simulink library "Uav_Electrical_lib"  (R2025a)
settings: Solver=ode23t  StartTime=0.0  StopTime=10  MaxStep=1e-3  RelTol=1e-3
values from neighbouring files (symbols this model uses):
  Ts = 2e-6    (= 2e-06)    [param.m]
undefined symbols (not defined in the file or in its folder): DiscIntNeverNeededParam, magnitude, uavParams
libraries: fl_lib x118, nesl_utility x61, spsCurrentMeasurementLib x23, spsIdealSwitchLib x12, spsVoltageMeasurementLib x11, simulink_extras x8, spsControlledCurrentSourceLib x7, spsSeriesRLCBranchLib x6, simulink x6, spsControlledVoltageSourceLib x5, spsPermanentMagnetSynchronousMachineLib x4, ee_lib x4
(part 2 of 5)

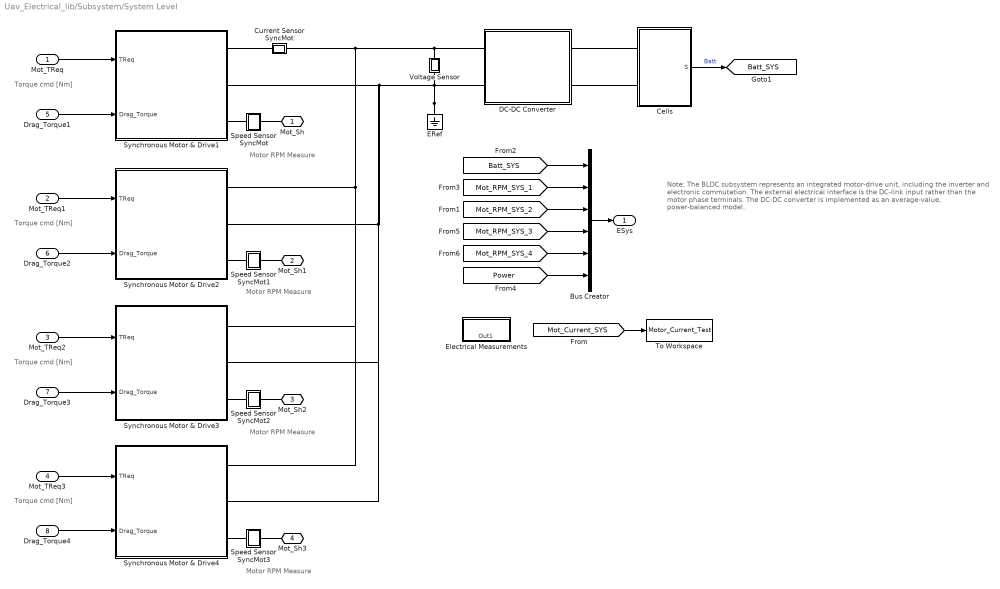
== system Uav_Electrical_lib/Subsystem/System Level ==
  note: Note:
      | The BLDC subsystem represents an integrated motor-drive unit, including the inverter and electronic commutation. The external electrical interface is the DC-link input rather than the motor phase terminals.
      |
      | The DC-DC converter is implemented as an average-value, power-balanced model.
  note: Motor RPM Measure
  note: Torque cmd [Nm]
  note: Motor RPM Measure
  note: Motor RPM Measure
  note: Motor RPM Measure
  note: Torque cmd [Nm]
  note: Torque cmd [Nm]
  note: Torque cmd [Nm]
  Mot_TReq : Inport
  Mot_TReq1 : Inport  Port=2
  Mot_TReq2 : Inport  Port=3
  Mot_TReq3 : Inport  Port=4
  Drag_Torque1 : Inport  Port=5
  Drag_Torque2 : Inport  Port=6
  Drag_Torque3 : Inport  Port=7
  Drag_Torque4 : Inport  Port=8
  Bus Creator : BusCreator  Inputs=6
  Cells : Subsystem
      mask Display:
      | port_label('LConn',1,'+');
      | port_label('LConn',2,'-');
      | port_label('output',1,'S');
  Current Sensor SyncMot : Subsystem
  DC-DC Converter : Subsystem  mask{Vout=uavParams.DCDCConv.Output_Voltage, RLoadLoss=uavParams.DCDCConv.Resistance_Losses, Kp=uavParams.DCDCConv.Kp, Ki=uavParams.DCDCConv.Ki}
      mask prompts: Vout "Output Voltage (V)"; RLoadLoss "Resistance, Load Dependent Losses (Ohm)"; Kp "Proportional Gain"; Ki "Integral Gain"
      mask Display:
      | port_label('RConn',1,'Bus+');
      | port_label('RConn',2,'Bus-');
      | port_label('LConn',1,'Batt+');
      | port_label('LConn',2,'Batt-');
      | text(0.05,0.5,'Out');
      | text(0.85,0.5,'In');
      | text(0.4,0.925,'Loss');
  ERef : fl_lib/Electrical/Electrical Elements/Electrical Reference
  Electrical Measurements : Subsystem
      settings: PortSchema="{\"entries\":[{\"content\":{\"sides\":[{\"content\":{},\"type\":\"ConnectorPlacement.EquallySpacedRectSide\",\"uuid\":\"d767dc0f-3242-457c-b485-d2cffe9a551f\"},{\"content\":{\"side\":\"RIGHT\"},\"type\":\"ConnectorPlacement.EquallySpacedRectSide\",\"uuid\":\"af281f4d-1d90-4252-9345-da5138a7006e\"},{\"content\":{\"side\":\"TOP\"},\"type\":\"ConnectorPlacement.EquallySpacedRectSide\",\"uuid\":\"dbc22d34-bfc6-4c39-8948-88a84cca37c4\"},{\"content\":{\"connectorIds\":[\"Out1\"],\"side\":\"BOTTOM\"},\"type\":\"ConnectorPlacement.EquallySpacedRectSide\",\"uuid\":\"dcc551d0-4ea4-47a9-a013-a7fbdb3e3c88\"}]},\"type\":\"ConnectorPlacement.EquallySpacedConnector\",\"uuid\":\"b183f40c-b7db-4954-8a30-0f5d22085f86\"}],\"packageUris\":[\"http://schema.mathworks.com/mf0/Connector/R2020b\"],\"version\":\"1.0\"}"
  Speed Sensor SyncMot : Subsystem
      mask Display: disp('S');
  Speed Sensor SyncMot1 : Subsystem
      mask Display: disp('S');
  Speed Sensor SyncMot2 : Subsystem
      mask Display: disp('S');
  Speed Sensor SyncMot3 : Subsystem
      mask Display: disp('S');
  Synchronous Motor & Drive1 : Subsystem
  Synchronous Motor & Drive2 : Subsystem
  Synchronous Motor & Drive3 : Subsystem
  Synchronous Motor & Drive4 : Subsystem
  To Workspace : ToWorkspace  VariableName=Motor_Current_Test  SaveFormat=Timeseries  SampleTime=-1
  Voltage Sensor : Subsystem
  Mot_Sh : PMIOPort  Side=Right
  Mot_Sh1 : PMIOPort  Port=2  Side=Right
  Mot_Sh2 : PMIOPort  Port=3  Side=Right
  Mot_Sh3 : PMIOPort  Port=4  Side=Right
  ESys : Outport  VectorParamsAs1DForOutWhenUnconnected=off
  tag scope: Batt_SYS=global
  wires:
  Bus Creator/1 -> ESys/1
  [Mot_RPM_SYS_1] -> Bus Creator/2
  Mot_TReq/1 -> Synchronous Motor & Drive1/1(TReq)
  Mot_TReq1/1 -> Synchronous Motor & Drive2/1(TReq)
  Mot_TReq2/1 -> Synchronous Motor & Drive3/1(TReq)
  Mot_TReq3/1 -> Synchronous Motor & Drive4/1(TReq)
  [Batt_SYS] -> Bus Creator/1
  Cells/1(S) -> [Batt_SYS]  "Batt"
  [Power] -> Bus Creator/6
  [Mot_RPM_SYS_4] -> Bus Creator/5
  [Mot_RPM_SYS_3] -> Bus Creator/4
  [Mot_RPM_SYS_2] -> Bus Creator/3
  [Mot_Current_SYS] -> To Workspace/1
  Drag_Torque1/1 -> Synchronous Motor & Drive1/2(Drag_Torque)
  Drag_Torque2/1 -> Synchronous Motor & Drive2/2(Drag_Torque)
  Drag_Torque3/1 -> Synchronous Motor & Drive3/2(Drag_Torque)
  Drag_Torque4/1 -> Synchronous Motor & Drive4/2(Drag_Torque)
  connections:
  Mot_Sh/RConn1 -- Speed Sensor SyncMot/RConn1
  Current Sensor SyncMot/RConn1 -- Synchronous Motor & Drive1/RConn1
  Speed Sensor SyncMot/LConn1 -- Synchronous Motor & Drive1/RConn3
  Mot_Sh1/RConn1 -- Speed Sensor SyncMot1/RConn1
  Synchronous Motor & Drive2/RConn3 -- Speed Sensor SyncMot1/LConn1
  Speed Sensor SyncMot2/LConn1 -- Synchronous Motor & Drive3/RConn3
  Mot_Sh2/RConn1 -- Speed Sensor SyncMot2/RConn1
  Mot_Sh3/RConn1 -- Speed Sensor SyncMot3/RConn1
  Speed Sensor SyncMot3/LConn1 -- Synchronous Motor & Drive4/RConn3
  Cells/LConn1 -- DC-DC Converter/LConn1
  Cells/LConn2 -- DC-DC Converter/LConn2
  Current Sensor SyncMot/LConn1 -- Synchronous Motor & Drive4/RConn1 -- Synchronous Motor & Drive3/RConn1 -- Synchronous Motor & Drive2/RConn1 -- DC-DC Converter/RConn1 -- Voltage Sensor/LConn1
  ERef/LConn1 -- Synchronous Motor & Drive3/RConn2 -- Synchronous Motor & Drive4/RConn2 -- Synchronous Motor & Drive2/RConn2 -- Synchronous Motor & Drive1/RConn2 -- DC-DC Converter/RConn2 -- Voltage Sensor/RConn1

== system Uav_Electrical_lib/Detailed （on-going work）/DC//DC Converter/PWM ==
  Ref. : Inport
  Data Type Conversion : DataTypeConversion
  Data Type Conversion1 : DataTypeConversion
  Mux : Mux  Inputs=2
  NOT : Logic  Operator=NOT  Inputs=1  AllPortsSameDT=off  OutDataTypeStr=uint(8)
  Rate Transition : RateTransition
  Relational Operator : RelationalOperator  Operator=>  InputSameDT=off
  Sawtooth generator : Subsystem
  Thermal Model : Subsystem
  Zero-Order Hold : ZeroOrderHold  SampleTime=Ts
  Pulses : Outport  VectorParamsAs1DForOutWhenUnconnected=off
  wires:
  NOT/1 -> Mux/2
  Rate Transition/1 -> Zero-Order Hold/1
  Relational Operator/1 -> Data Type Conversion/1
  Data Type Conversion/1 -> Mux/1, NOT/1
  Zero-Order Hold/1 -> Relational Operator/1
  Sawtooth generator/1(Out) -> Relational Operator/2
  Ref./1 -> Rate Transition/1, Thermal Model/1(IBus)
  Mux/1 -> Data Type Conversion1/1
  Data Type Conversion1/1 -> Pulses/1

== system Uav_Electrical_lib/Detailed （on-going work）/DC//DC Converter/Voltage Controller ==
  Uref : Inport
  UBus : Inport  Port=2
  Clock1 : Clock
  Compare To Constant1 : simulink/Logic and Bit Operations/Compare To Constant  relop=>  const=0.01  OutDataTypeStr=uint8  ZeroCross=off
  Ctrl sat. : Saturate  UpperLimit=0.95  LowerLimit=-0.95
  Discrete-Time Integrator : DiscreteIntegrator  IntegratorMethod=Integration: Trapezoidal  SampleTime=Ts  LimitOutput=on  UpperSaturationLimit=1  LowerSaturationLimit=-1  ICPrevOutput=DiscIntNeverNeededParam  ICPrevScaledInput=DiscIntNeverNeededParam
  Integral gain : Gain  Gain=Ki  SaturateOnIntegerOverflow=on  OutDataTypeStr=Inherit: Same as input  ParamDataTypeStr=Inherit: Same as input
  Product1 : Product  RndMeth=Zero
  Proportional gain : Gain  Gain=Kp  SaturateOnIntegerOverflow=on  OutDataTypeStr=Inherit: Same as input  ParamDataTypeStr=Inherit: Same as input
  Sum1 : Sum  Inputs=+-  InputSameDT=on  SaturateOnIntegerOverflow=on  OutDataTypeStr=Inherit: Same as first input
  Sum2 : Sum  InputSameDT=on  SaturateOnIntegerOverflow=on  OutDataTypeStr=Inherit: Same as first input
  Transfer Fcn : TransferFcn  Denominator=[.0001 1]
  Zero-Order Hold1 : ZeroOrderHold  SampleTime=Ts
  Ec : Outport  InitialOutput=0  VectorParamsAs1DForOutWhenUnconnected=off
  wires:
  Sum2/1 -> Ctrl sat./1
  Discrete-Time Integrator/1 -> Sum2/2
  UBus/1 -> Zero-Order Hold1/1
  Integral gain/1 -> Discrete-Time Integrator/1
  Proportional gain/1 -> Sum2/1
  Ctrl sat./1 -> Ec/1
  Sum1/1 -> Product1/1
  Clock1/1 -> Compare To Constant1/1
  Compare To Constant1/1 -> Product1/2
  Product1/1 -> Integral gain/1, Proportional gain/1
  Zero-Order Hold1/1 -> Transfer Fcn/1
  Transfer Fcn/1 -> Sum1/1
  Uref/1 -> Sum1/2

== system Uav_Electrical_lib/Detailed （on-going work）/Synchronous Generator & Drive/GF ==
  In1 : Inport
  Out1 : Outport  VectorParamsAs1DForOutWhenUnconnected=off
  tag scope: Gen_TReq_SYS=global
  wires:
  In1/1 -> Out1/1, [Gen_TReq_SYS]

== system Uav_Electrical_lib/Detailed （on-going work）/Synchronous Generator & Drive/Measures ==
  Current Measurement : spsCurrentMeasurementLib/Current Measurement  Tag=PoWeRsYsTeMmEaSuReMeNt  PhasorSimulation=off  OutputType=Magnitude  PSBequivalent=0
      settings: AttributesFormatString=\n
  Current Measurement1 : spsCurrentMeasurementLib/Current Measurement  Tag=PoWeRsYsTeMmEaSuReMeNt  PhasorSimulation=off  OutputType=Magnitude  PSBequivalent=0
      settings: AttributesFormatString=\n
  Current Measurement2 : spsCurrentMeasurementLib/Current Measurement  Tag=PoWeRsYsTeMmEaSuReMeNt  PhasorSimulation=off  OutputType=Magnitude  PSBequivalent=0
      settings: AttributesFormatString=\n
  Mux1 : Mux  Inputs=3
  Ta : PMIOPort  Side=Left
  Tb : PMIOPort  Port=2  Side=Left
  Tc : PMIOPort  Port=3  Side=Left
  Mta : PMIOPort  Port=4  Side=Right
  Mtb : PMIOPort  Port=5  Side=Right
  Mtc : PMIOPort  Port=6  Side=Right
  I_abc : Outport  VectorParamsAs1DForOutWhenUnconnected=off
  wires:
  Current Measurement1/1 -> Mux1/2
  Current Measurement/1 -> Mux1/1
  Current Measurement2/1 -> Mux1/3
  Mux1/1 -> I_abc/1
  connections:
  Current Measurement1/RConn1 -- Mtb/RConn1
  Tb/RConn1 -- Current Measurement1/LConn1
  Current Measurement/RConn1 -- Mta/RConn1
  Ta/RConn1 -- Current Measurement/LConn1
  Tc/RConn1 -- Current Measurement2/LConn1
  Current Measurement2/RConn1 -- Mtc/RConn1

== system Uav_Electrical_lib/Detailed （on-going work）/Synchronous Generator & Drive/Mux ==
  gates : Inport
  m : Inport  Port=2
  Terminator : Terminator
  g : Outport  VectorParamsAs1DForOutWhenUnconnected=off
  wires:
  gates/1 -> g/1
  m/1 -> Terminator/1

== system Uav_Electrical_lib/Detailed （on-going work）/Synchronous Generator & Drive/Subsystem ==
  In : Inport
  "+ -> -1" : Gain  Gain=30/pi
  Bus Selector : BusSelector  OutputSignals=Stator current is_a (A),Rotor speed wm (rad/s),Electromagnetic torque Te (N*m)
  Mux1 : Mux  Inputs=2
  Mux2 : Mux  Inputs=3
  Out : Outport  VectorParamsAs1DForOutWhenUnconnected=off
  tag scope: GeneratorDrive=global
  wires:
  In/1 -> Bus Selector/1, Out/1
  "+ -> -1"/1 -> Mux2/2
  [Gen_TReq_SYS] -> Mux1/2
  Bus Selector/2 -> "+ -> -1"/1  "<Rotor speed wm (rad/s)>"
  Bus Selector/3 -> Mux1/1  "<Electromagnetic torque Te (N*m)>"
  Mux1/1 -> Mux2/3
  Bus Selector/1 -> Mux2/1  "<Stator current is_a (A)>"
  Mux2/1 -> [GeneratorDrive]

== system Uav_Electrical_lib/Detailed （on-going work）/Synchronous Generator & Drive/Subsystem1 ==
  Sig : Inport
  Bus Selector : BusSelector  OutputSignals=Electromagnetic torque Te (N*m)
  Ideal Rotational Motion Sensor : fl_lib/Mechanical/Mechanical Sensors/Ideal Rotational Motion Sensor  reference=foundation.enum.MeasurementReference.difference  acceleration_port=false  velocity_port=true  position_port=true  wrap_angle=simscape.enum.onoff.off  offset=0 rad
  Ideal Torque Source : fl_lib/Mechanical/Mechanical Sources/Ideal Torque Source
  Mechanical Rotational Reference : fl_lib/Mechanical/Rotational Elements/Mechanical Rotational Reference
  Mechanical Rotational Reference1 : fl_lib/Mechanical/Rotational Elements/Mechanical Rotational Reference
  PS-Simulink Converter : nesl_utility/PS-Simulink Converter  PhysicalDomain=network_engine_domain  SubClassName=ps_output  LeftPortType=input  RightPortType=output  PseudoPeriodic=off  Frequencies=[]  VectorFormat=1-D array  Unit=rad/s  AffineConversion=off
  Simulink-PS Converter : nesl_utility/Simulink-PS Converter  PhysicalDomain=network_engine_domain  SubClassName=ps_input  LeftPortType=input  RightPortType=output  PseudoPeriodic=off  Frequencies=[]  NoiseDistribution=none  NoiseParameters=[]  Unit=1  AffineConversion=off  FilteringAndDerivatives=zero  SimscapeFilterOrder=1  InputFilterTimeConstant=0.005  UdotUserProvided=0
  Sh : PMIOPort  Side=Right
  Spd : Outport  VectorParamsAs1DForOutWhenUnconnected=off
  wires:
  Bus Selector/1 -> Simulink-PS Converter/1  "<Electromagnetic torque Te (N*m)>"
  Sig/1 -> Bus Selector/1
  PS-Simulink Converter/1 -> Spd/1
  connections:
  Mechanical Rotational Reference/LConn1 -- Ideal Rotational Motion Sensor/RConn1
  Mechanical Rotational Reference1/LConn1 -- Ideal Torque Source/RConn2
  Ideal Torque Source/LConn1 -- Sh/RConn1 -- Ideal Rotational Motion Sensor/LConn1
  PS-Simulink Converter/LConn1 -- Ideal Rotational Motion Sensor/RConn2
  Simulink-PS Converter/RConn1 -- Ideal Torque Source/RConn1

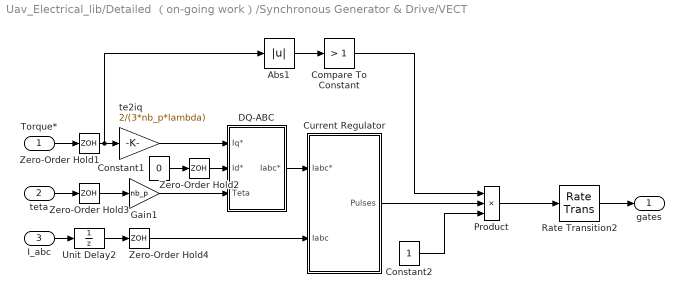
== system Uav_Electrical_lib/Detailed （on-going work）/Synchronous Generator & Drive/VECT ==
  Torque* : Inport
  teta : Inport  Port=2
  I_abc : Inport  Port=3
  Abs1 : Abs  SaturateOnIntegerOverflow=off
  Compare To Constant : simulink/Logic and Bit Operations/Compare To Constant  relop=>  const=1  OutDataTypeStr=uint8
  Constant1 : Constant  Value=0
  Constant2 : Constant
  Current Regulator : Subsystem
  DQ-ABC : Subsystem
  Gain1 : Gain  Gain=nb_p  SaturateOnIntegerOverflow=on  OutDataTypeStr=Inherit: Same as input  ParamDataTypeStr=Inherit: Same as input
  Product : Product  Inputs=3  RndMeth=Zero
  Rate Transition2 : RateTransition
  Unit Delay2 : UnitDelay  SampleTime=-1  HasFrameUpgradeWarning=on
  Zero-Order Hold{1..4} (4 alike) : ZeroOrderHold  SampleTime=Ts_vect
  te2iq : Gain  Gain=2/(3*nb_p*lambda)  SaturateOnIntegerOverflow=on  OutDataTypeStr=Inherit: Same as input  ParamDataTypeStr=Inherit: Same as input
  gates : Outport  VectorParamsAs1DForOutWhenUnconnected=off
  wires:
  Compare To Constant/1 -> Product/1
  Abs1/1 -> Compare To Constant/1
  Constant2/1 -> Product/3
  I_abc/1 -> Unit Delay2/1
  DQ-ABC/1(Iabc*) -> Current Regulator/1(Iabc*)
  Gain1/1 -> DQ-ABC/3(Teta)
  Constant1/1 -> Zero-Order Hold2/1
  Torque*/1 -> Zero-Order Hold1/1
  Zero-Order Hold3/1 -> Gain1/1
  teta/1 -> Zero-Order Hold3/1
  Current Regulator/1(Pulses) -> Product/2
  Zero-Order Hold1/1 -> Abs1/1, te2iq/1
  Zero-Order Hold4/1 -> Current Regulator/2(Iabc)
  Zero-Order Hold2/1 -> DQ-ABC/2("Id* ")
  Rate Transition2/1 -> gates/1
  Product/1 -> Rate Transition2/1
  te2iq/1 -> DQ-ABC/1("Iq* ")
  Unit Delay2/1 -> Zero-Order Hold4/1

== system Uav_Electrical_lib/Detailed （on-going work）/Synchronous Motor & Drive/GF ==
  In1 : Inport
  Out1 : Outport  VectorParamsAs1DForOutWhenUnconnected=off
  tag scope: Mot_TReq_SYS=global
  wires:
  In1/1 -> Out1/1, [Mot_TReq_SYS]

== system Uav_Electrical_lib/Detailed （on-going work）/Synchronous Motor & Drive/Measures ==
  Current Measurement : spsCurrentMeasurementLib/Current Measurement  Tag=PoWeRsYsTeMmEaSuReMeNt  PhasorSimulation=off  OutputType=Magnitude  PSBequivalent=0
      settings: AttributesFormatString=\n
  Current Measurement1 : spsCurrentMeasurementLib/Current Measurement  Tag=PoWeRsYsTeMmEaSuReMeNt  PhasorSimulation=off  OutputType=Magnitude  PSBequivalent=0
      settings: AttributesFormatString=\n
  Current Measurement2 : spsCurrentMeasurementLib/Current Measurement  Tag=PoWeRsYsTeMmEaSuReMeNt  PhasorSimulation=off  OutputType=Magnitude  PSBequivalent=0
      settings: AttributesFormatString=\n
  Mux1 : Mux  Inputs=3
  Ta : PMIOPort  Side=Left
  Tb : PMIOPort  Port=2  Side=Left
  Tc : PMIOPort  Port=3  Side=Left
  Mta : PMIOPort  Port=4  Side=Right
  Mtb : PMIOPort  Port=5  Side=Right
  Mtc : PMIOPort  Port=6  Side=Right
  I_abc : Outport  VectorParamsAs1DForOutWhenUnconnected=off
  wires:
  Current Measurement1/1 -> Mux1/2
  Current Measurement/1 -> Mux1/1
  Current Measurement2/1 -> Mux1/3
  Mux1/1 -> I_abc/1
  connections:
  Current Measurement1/RConn1 -- Mtb/RConn1
  Tb/RConn1 -- Current Measurement1/LConn1
  Current Measurement/RConn1 -- Mta/RConn1
  Ta/RConn1 -- Current Measurement/LConn1
  Tc/RConn1 -- Current Measurement2/LConn1
  Current Measurement2/RConn1 -- Mtc/RConn1

== system Uav_Electrical_lib/Detailed （on-going work）/Synchronous Motor & Drive/Mux ==
  gates : Inport
  m : Inport  Port=2
  Terminator : Terminator
  g : Outport  VectorParamsAs1DForOutWhenUnconnected=off
  wires:
  m/1 -> Terminator/1
  gates/1 -> g/1

== system Uav_Electrical_lib/Detailed （on-going work）/Synchronous Motor & Drive/Subsystem ==
  In : Inport
  "+ -> -1" : Gain  Gain=30/pi
  Bus Selector : BusSelector  OutputSignals=Stator current is_a (A),Rotor speed wm (rad/s),Electromagnetic torque Te (N*m)
  Mux1 : Mux  Inputs=2
  Mux2 : Mux  Inputs=3
  Out : Outport  VectorParamsAs1DForOutWhenUnconnected=off
  tag scope: MotorDrive=global
  wires:
  In/1 -> Bus Selector/1, Out/1
  "+ -> -1"/1 -> Mux2/2
  [Mot_TReq_SYS] -> Mux1/2
  Bus Selector/2 -> "+ -> -1"/1  "<Rotor speed wm (rad/s)>"
  Bus Selector/3 -> Mux1/1  "<Electromagnetic torque Te (N*m)>"
  Mux1/1 -> Mux2/3
  Bus Selector/1 -> Mux2/1  "<Stator current is_a (A)>"
  Mux2/1 -> [MotorDrive]

== system Uav_Electrical_lib/Detailed （on-going work）/Synchronous Motor & Drive/Subsystem1 ==
  Sig : Inport
  Bus Selector : BusSelector  OutputSignals=Electromagnetic torque Te (N*m)
  Ideal Rotational Motion Sensor : fl_lib/Mechanical/Mechanical Sensors/Ideal Rotational Motion Sensor  reference=foundation.enum.MeasurementReference.difference  acceleration_port=false  velocity_port=true  position_port=true  wrap_angle=simscape.enum.onoff.off  offset=0 rad
  Ideal Torque Source : fl_lib/Mechanical/Mechanical Sources/Ideal Torque Source
  Mechanical Rotational Reference : fl_lib/Mechanical/Rotational Elements/Mechanical Rotational Reference
  Mechanical Rotational Reference1 : fl_lib/Mechanical/Rotational Elements/Mechanical Rotational Reference
  PS-Simulink Converter : nesl_utility/PS-Simulink Converter  PhysicalDomain=network_engine_domain  SubClassName=ps_output  LeftPortType=input  RightPortType=output  PseudoPeriodic=off  Frequencies=[]  VectorFormat=1-D array  Unit=rad/s  AffineConversion=off
  Simulink-PS Converter : nesl_utility/Simulink-PS Converter  PhysicalDomain=network_engine_domain  SubClassName=ps_input  LeftPortType=input  RightPortType=output  PseudoPeriodic=off  Frequencies=[]  NoiseDistribution=none  NoiseParameters=[]  Unit=1  AffineConversion=off  FilteringAndDerivatives=zero  SimscapeFilterOrder=1  InputFilterTimeConstant=0.005  UdotUserProvided=0
  Sh : PMIOPort  Side=Right
  Spd : Outport  VectorParamsAs1DForOutWhenUnconnected=off
  wires:
  PS-Simulink Converter/1 -> Spd/1
  Sig/1 -> Bus Selector/1
  Bus Selector/1 -> Simulink-PS Converter/1  "<Electromagnetic torque Te (N*m)>"
  connections:
  Simulink-PS Converter/RConn1 -- Ideal Torque Source/RConn1
  PS-Simulink Converter/LConn1 -- Ideal Rotational Motion Sensor/RConn2
  Ideal Rotational Motion Sensor/LConn1 -- Sh/RConn1 -- Ideal Torque Source/LConn1
  Mechanical Rotational Reference1/LConn1 -- Ideal Torque Source/RConn2
  Mechanical Rotational Reference/LConn1 -- Ideal Rotational Motion Sensor/RConn1

== system Uav_Electrical_lib/Detailed （on-going work）/Synchronous Motor & Drive/Torque limitation ==
  N rad/s : Inport
  Torque : Inport  Port=2
  Abs1 : Abs
  Gain : Gain  Gain=-1
  Saturation Dynamic : simulink/Discontinuities/Saturation Dynamic  OutMin=[]  OutMax=[]  OutDataTypeStr=Inherit: Same as second input  OutDataType=sfix(16)  OutScaling=2^-10  DoSatur=off
  Torque vs speed profile : Lookup  InputValues=[0 1200 2000 3000 4000 5000 6000]*pi/30  Table=[400 400 225 150 100 80 70]  SaturateOnIntegerOverflow=off
  torque : Outport  VectorParamsAs1DForOutWhenUnconnected=off
  wires:
  Gain/1 -> Saturation Dynamic/3
  Torque/1 -> Saturation Dynamic/2
  Saturation Dynamic/1 -> torque/1
  Torque vs speed profile/1 -> Gain/1, Saturation Dynamic/1
  Abs1/1 -> Torque vs speed profile/1
  N rad/s/1 -> Abs1/1

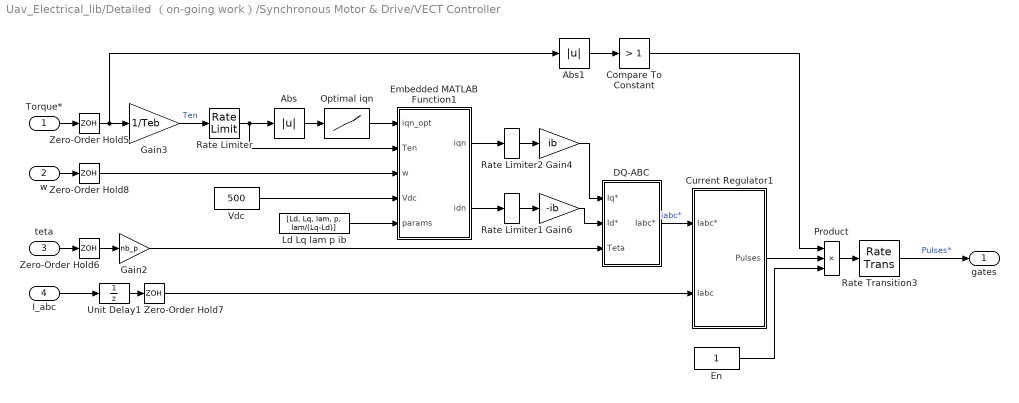
== system Uav_Electrical_lib/Detailed （on-going work）/Synchronous Motor & Drive/VECT Controller ==
  Torque* : Inport
  w : Inport  Port=2
  teta : Inport  Port=3
  I_abc : Inport  Port=4
  Abs : Abs  SaturateOnIntegerOverflow=off
  Abs1 : Abs  SaturateOnIntegerOverflow=off
  Compare To Constant : simulink/Logic and Bit Operations/Compare To Constant  relop=>  const=1  OutDataTypeStr=uint8
  Current Regulator1 : Subsystem
  DQ-ABC : Subsystem
  Embedded MATLAB Function1 : MATLAB Function  TreatAsAtomicUnit=on  SystemSampleTime=Ts_vect
  En : Constant
  Gain2 : Gain  Gain=nb_p  SaturateOnIntegerOverflow=on  OutDataTypeStr=Inherit: Same as input  ParamDataTypeStr=Inherit: Same as input
  Gain3 : Gain  Gain=1/Teb  SaturateOnIntegerOverflow=on  OutDataTypeStr=Inherit: Same as input  ParamDataTypeStr=Inherit: Same as input
  Gain4 : Gain  Gain=ib  SaturateOnIntegerOverflow=on  OutDataTypeStr=Inherit: Same as input  ParamDataTypeStr=Inherit: Same as input
  Gain6 : Gain  Gain=-ib  SaturateOnIntegerOverflow=on  OutDataTypeStr=Inherit: Same as input  ParamDataTypeStr=Inherit: Same as input
  Ld Lq lam p ib : Constant  Value=[Ld, Lq, lam, p, lam/(Lq-Ld)]
  Optimal iqn : Lookup  InputValues=ten  Table=iqn  SaturateOnIntegerOverflow=off
  Product : Product  Inputs=3  RndMeth=Zero
  Rate Limiter : RateLimiter  RisingSlewLimit=10  FallingSlewLimit=-10  LinearizeAsGain=off
  Rate Limiter1 : RateLimiter  RisingSlewLimit=100  FallingSlewLimit=-100  SampleTimeMode=inherited
  Rate Limiter2 : RateLimiter  RisingSlewLimit=100  FallingSlewLimit=-100  SampleTimeMode=inherited
  Rate Transition3 : RateTransition
  Unit Delay1 : UnitDelay  SampleTime=-1  HasFrameUpgradeWarning=on
  Vdc : Constant  Value=500
  Zero-Order Hold{5..8} (4 alike) : ZeroOrderHold  SampleTime=Ts_vect
  gates : Outport  VectorParamsAs1DForOutWhenUnconnected=off
  wires:
  Abs1/1 -> Compare To Constant/1
  Compare To Constant/1 -> Product/1
  En/1 -> Product/3
  Current Regulator1/1(Pulses) -> Product/2
  Unit Delay1/1 -> Zero-Order Hold7/1
  Zero-Order Hold7/1 -> Current Regulator1/2(Iabc)
  teta/1 -> Zero-Order Hold6/1
  Zero-Order Hold6/1 -> Gain2/1
  Gain2/1 -> DQ-ABC/3(Teta)
  DQ-ABC/1(Iabc*) -> Current Regulator1/1(Iabc*)  "iabc*"
  I_abc/1 -> Unit Delay1/1
  Torque*/1 -> Zero-Order Hold5/1
  Gain4/1 -> DQ-ABC/1("Iq* ")
  Gain6/1 -> DQ-ABC/2("Id* ")
  Zero-Order Hold5/1 -> Abs1/1, Gain3/1
  w/1 -> Zero-Order Hold8/1
  Embedded MATLAB Function1/2(idn) -> Rate Limiter1/1
  Gain3/1 -> Rate Limiter/1  "Ten"
  Zero-Order Hold8/1 -> Embedded MATLAB Function1/3(w)
  Ld Lq lam p ib/1 -> Embedded MATLAB Function1/5(params)
  Embedded MATLAB Function1/1(iqn) -> Rate Limiter2/1
  Optimal iqn/1 -> Embedded MATLAB Function1/1(iqn_opt)
  Abs/1 -> Optimal iqn/1
  Vdc/1 -> Embedded MATLAB Function1/4(Vdc)
  Rate Transition3/1 -> gates/1  "Pulses*"
  Product/1 -> Rate Transition3/1
  Rate Limiter2/1 -> Gain4/1
  Rate Limiter1/1 -> Gain6/1
  Rate Limiter/1 -> Abs/1, Embedded MATLAB Function1/2(Ten)

== system Uav_Electrical_lib/Mean Value（on-going work）/DC//DC Converter/Boost Converter Average-Values ==
  Duty Cycle : Inport
  Average-value armature voltage : Fcn  Expr=u(1)*u(2)
  Average-value source current : Fcn  Expr=u(1)*u(2)
  Controlled Current Source : spsControlledCurrentSourceLib/Controlled Current Source  Initialize=on  Source_Type=AC  Amplitude=0  Phase=0  Frequency=0  Measurements=None
  Controlled Voltage Source : spsControlledVoltageSourceLib/Controlled Voltage Source  Initialize=on  Source_Type=AC  Amplitude=0  Phase=0  Frequency=0  Measurements=None
  Current Measurement : spsCurrentMeasurementLib/Current Measurement  Tag=PoWeRsYsTeMmEaSuReMeNt  PhasorSimulation=off  OutputType=Magnitude  PSBequivalent=0
      settings: AttributesFormatString=\n
  Mux : Mux  Inputs=2
  Mux1 : Mux  Inputs=2
  Selector : Selector  InputPortWidth=2  IndexOptions=Index vector (dialog)  Indices=[1]  OutputSizes=1
  Thermal Model : Subsystem
  Unit Delay : UnitDelay  SampleTime=Ts  HasFrameUpgradeWarning=on
  Unit Delay1 : UnitDelay  SampleTime=Ts  HasFrameUpgradeWarning=on
  Voltage Measurement1 : spsVoltageMeasurementLib/Voltage Measurement  Tag=PoWeRsYsTeMmEaSuReMeNt  PhasorSimulation=off  OutputType=Magnitude  PSBequivalent=0
  A : PMIOPort  Side=Right
  + : PMIOPort  Port=2  Side=Left
  - : PMIOPort  Port=3  Side=Left
  wires:
  Unit Delay/1 -> Controlled Voltage Source/1
  Average-value armature voltage/1 -> Unit Delay/1
  Mux/1 -> Average-value armature voltage/1
  Voltage Measurement1/1 -> Mux/2
  Duty Cycle/1 -> Selector/1
  Mux1/1 -> Average-value source current/1
  Current Measurement/1 -> Mux1/2
  Average-value source current/1 -> Unit Delay1/1
  Unit Delay1/1 -> Controlled Current Source/1, Thermal Model/1(IBus)
  Selector/1 -> Mux/1, Mux1/1
  connections:
  Voltage Measurement1/LConn2 -- Controlled Current Source/RConn1 -- -/RConn1 -- Controlled Voltage Source/LConn1
  Controlled Current Source/LConn1 -- Voltage Measurement1/LConn1 -- +/RConn1
  Controlled Voltage Source/RConn1 -- Current Measurement/LConn1
  A/RConn1 -- Current Measurement/RConn1

== system Uav_Electrical_lib/Mean Value（on-going work）/DC//DC Converter/Current controller DISCRETE3 ==
  Uref : Inport
  UBus : Inport  Port=2
  Clock1 : Clock
  Compare To Constant1 : simulink/Logic and Bit Operations/Compare To Constant  relop=>  const=0.01  OutDataTypeStr=uint8  ZeroCross=off
  Ctrl sat. : Saturate  UpperLimit=0.95  LowerLimit=-0.95
  Discrete-Time Integrator : DiscreteIntegrator  IntegratorMethod=Integration: Trapezoidal  SampleTime=Ts  LimitOutput=on  UpperSaturationLimit=1  LowerSaturationLimit=-1  ICPrevOutput=DiscIntNeverNeededParam  ICPrevScaledInput=DiscIntNeverNeededParam
  Integral gain : Gain  Gain=Ki  SaturateOnIntegerOverflow=on  OutDataTypeStr=Inherit: Same as input  ParamDataTypeStr=Inherit: Same as input
  Product1 : Product  RndMeth=Zero
  Proportional gain : Gain  Gain=Kp  SaturateOnIntegerOverflow=on  OutDataTypeStr=Inherit: Same as input  ParamDataTypeStr=Inherit: Same as input
  Sum1 : Sum  Inputs=+-  InputSameDT=on  SaturateOnIntegerOverflow=on  OutDataTypeStr=Inherit: Same as first input
  Sum2 : Sum  InputSameDT=on  SaturateOnIntegerOverflow=on  OutDataTypeStr=Inherit: Same as first input
  Transfer Fcn : TransferFcn  Denominator=[.0001 1]
  Zero-Order Hold1 : ZeroOrderHold  SampleTime=Ts
  Ec : Outport  InitialOutput=0  VectorParamsAs1DForOutWhenUnconnected=off
  wires:
  Sum2/1 -> Ctrl sat./1
  Discrete-Time Integrator/1 -> Sum2/2
  UBus/1 -> Zero-Order Hold1/1
  Integral gain/1 -> Discrete-Time Integrator/1
  Proportional gain/1 -> Sum2/1
  Ctrl sat./1 -> Ec/1
  Sum1/1 -> Product1/1
  Clock1/1 -> Compare To Constant1/1
  Compare To Constant1/1 -> Product1/2
  Product1/1 -> Integral gain/1, Proportional gain/1
  Zero-Order Hold1/1 -> Transfer Fcn/1
  Transfer Fcn/1 -> Sum1/1
  Uref/1 -> Sum1/2

== system Uav_Electrical_lib/Mean Value（on-going work）/DC//DC Converter/Duty Cycles ==
  Ec : Inport
  Add : Sum  Inputs=+-
  Bus Creator2 : BusCreator  Inputs=2
  Constant : Constant
  Duty Cycle : Fcn  Expr=0.5*(u[1]+1)
  Unit Delay2 : UnitDelay  InitialCondition=.5  SampleTime=Ts  HasFrameUpgradeWarning=on
  dc : Outport  VectorParamsAs1DForOutWhenUnconnected=off
  wires:
  Bus Creator2/1 -> Unit Delay2/1
  Ec/1 -> Duty Cycle/1
  Constant/1 -> Add/1
  Add/1 -> Bus Creator2/2  "IGBT 2"
  Duty Cycle/1 -> Bus Creator2/1, Add/2  "IGBT I"
  Unit Delay2/1 -> dc/1

== system Uav_Electrical_lib/Mean Value（on-going work）/Synchronous Generator & Drive/GF ==
  In1 : Inport
  Out1 : Outport  VectorParamsAs1DForOutWhenUnconnected=off
  tag scope: Gen_TReq_SYS=global
  wires:
  In1/1 -> Out1/1, [Gen_TReq_SYS]

== system Uav_Electrical_lib/Mean Value（on-going work）/Synchronous Generator & Drive/Measures ==
  Current Measurement : spsCurrentMeasurementLib/Current Measurement  Tag=PoWeRsYsTeMmEaSuReMeNt  PhasorSimulation=off  OutputType=Magnitude  PSBequivalent=0
      settings: AttributesFormatString=\n
  Current Measurement1 : spsCurrentMeasurementLib/Current Measurement  Tag=PoWeRsYsTeMmEaSuReMeNt  PhasorSimulation=off  OutputType=Magnitude  PSBequivalent=0
      settings: AttributesFormatString=\n
  Current Measurement2 : spsCurrentMeasurementLib/Current Measurement  Tag=PoWeRsYsTeMmEaSuReMeNt  PhasorSimulation=off  OutputType=Magnitude  PSBequivalent=0
      settings: AttributesFormatString=\n
  Mux1 : Mux  Inputs=3
  Ta : PMIOPort  Side=Left
  Tb : PMIOPort  Port=2  Side=Left
  Tc : PMIOPort  Port=3  Side=Left
  Mta : PMIOPort  Port=4  Side=Right
  Mtb : PMIOPort  Port=5  Side=Right
  Mtc : PMIOPort  Port=6  Side=Right
  I_abc : Outport  VectorParamsAs1DForOutWhenUnconnected=off
  wires:
  Current Measurement1/1 -> Mux1/2
  Current Measurement/1 -> Mux1/1
  Current Measurement2/1 -> Mux1/3
  Mux1/1 -> I_abc/1
  connections:
  Current Measurement1/RConn1 -- Mtb/RConn1
  Tb/RConn1 -- Current Measurement1/LConn1
  Current Measurement/RConn1 -- Mta/RConn1
  Ta/RConn1 -- Current Measurement/LConn1
  Tc/RConn1 -- Current Measurement2/LConn1
  Current Measurement2/RConn1 -- Mtc/RConn1

== system Uav_Electrical_lib/Mean Value（on-going work）/Synchronous Generator & Drive/Mux ==
  sig* : Inport
  m : Inport  Port=2
  Bus Creator : BusCreator  Inputs=2
  Ctrl : Outport  VectorParamsAs1DForOutWhenUnconnected=off
  wires:
  Bus Creator/1 -> Ctrl/1
  sig*/1 -> Bus Creator/1  "Signals*"
  m/1 -> Bus Creator/2  "m"

== system Uav_Electrical_lib/Mean Value（on-going work）/Synchronous Generator & Drive/Subsystem ==
  In : Inport
  "+ -> -1" : Gain  Gain=30/pi
  Bus Selector : BusSelector  OutputSignals=Stator current is_a (A),Rotor speed wm (rad/s),Electromagnetic torque Te (N*m)
  Mux1 : Mux  Inputs=2
  Mux2 : Mux  Inputs=3
  Out : Outport  VectorParamsAs1DForOutWhenUnconnected=off
  tag scope: GeneratorDrive=global
  wires:
  In/1 -> Bus Selector/1, Out/1
  "+ -> -1"/1 -> Mux2/2
  [Gen_TReq_SYS] -> Mux1/2
  Bus Selector/2 -> "+ -> -1"/1  "<Rotor speed wm (rad/s)>"
  Bus Selector/3 -> Mux1/1  "<Electromagnetic torque Te (N*m)>"
  Mux1/1 -> Mux2/3
  Bus Selector/1 -> Mux2/1  "<Stator current is_a (A)>"
  Mux2/1 -> [GeneratorDrive]

== system Uav_Electrical_lib/Mean Value（on-going work）/Synchronous Generator & Drive/Subsystem1 ==
  Sig : Inport
  Bus Selector : BusSelector  OutputSignals=Electromagnetic torque Te (N*m)
  Ideal Rotational Motion Sensor : fl_lib/Mechanical/Mechanical Sensors/Ideal Rotational Motion Sensor  reference=foundation.enum.MeasurementReference.difference  acceleration_port=false  velocity_port=true  position_port=true  wrap_angle=simscape.enum.onoff.off  offset=0 rad
  Ideal Torque Source : fl_lib/Mechanical/Mechanical Sources/Ideal Torque Source
  Mechanical Rotational Reference : fl_lib/Mechanical/Rotational Elements/Mechanical Rotational Reference
  Mechanical Rotational Reference1 : fl_lib/Mechanical/Rotational Elements/Mechanical Rotational Reference
  PS-Simulink Converter : nesl_utility/PS-Simulink Converter  PhysicalDomain=network_engine_domain  SubClassName=ps_output  LeftPortType=input  RightPortType=output  PseudoPeriodic=off  Frequencies=[]  VectorFormat=1-D array  Unit=rad/s  AffineConversion=off
  Simulink-PS Converter : nesl_utility/Simulink-PS Converter  PhysicalDomain=network_engine_domain  SubClassName=ps_input  LeftPortType=input  RightPortType=output  PseudoPeriodic=off  Frequencies=[]  NoiseDistribution=none  NoiseParameters=[]  Unit=1  AffineConversion=off  FilteringAndDerivatives=zero  SimscapeFilterOrder=1  InputFilterTimeConstant=0.005  UdotUserProvided=0
  Sh : PMIOPort  Side=Right
  Spd : Outport  VectorParamsAs1DForOutWhenUnconnected=off
  wires:
  PS-Simulink Converter/1 -> Spd/1
  Sig/1 -> Bus Selector/1
  Bus Selector/1 -> Simulink-PS Converter/1  "<Electromagnetic torque Te (N*m)>"
  connections:
  Simulink-PS Converter/RConn1 -- Ideal Torque Source/RConn1
  PS-Simulink Converter/LConn1 -- Ideal Rotational Motion Sensor/RConn2
  Ideal Rotational Motion Sensor/LConn1 -- Sh/RConn1 -- Ideal Torque Source/LConn1
  Mechanical Rotational Reference1/LConn1 -- Ideal Torque Source/RConn2
  Mechanical Rotational Reference/LConn1 -- Ideal Rotational Motion Sensor/RConn1

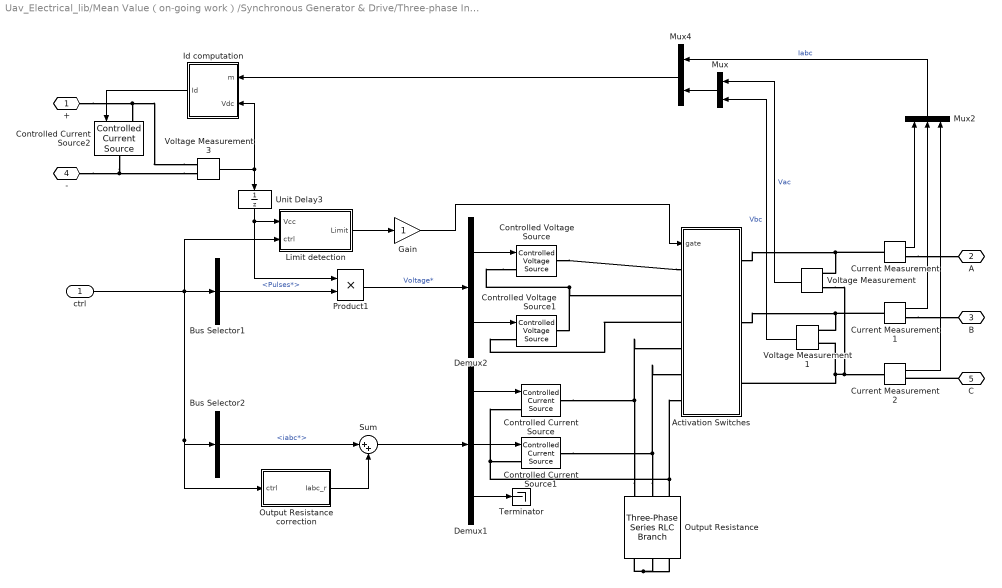
== system Uav_Electrical_lib/Mean Value（on-going work）/Synchronous Generator & Drive/Three-phase Inverter ==
  ctrl : Inport
  Activation Switches : Subsystem
  Bus Selector1 : BusSelector  OutputSignals=Signals*.Pulses*
  Bus Selector2 : BusSelector  OutputSignals=Signals*.iabc*
  Controlled Current Source : spsControlledCurrentSourceLib/Controlled Current Source  Initialize=on  Source_Type=AC  Amplitude=0  Phase=0  Frequency=0  Measurements=None
  Controlled Current Source1 : spsControlledCurrentSourceLib/Controlled Current Source  Initialize=on  Source_Type=AC  Amplitude=0  Phase=0  Frequency=0  Measurements=None
  Controlled Current Source2 : spsControlledCurrentSourceLib/Controlled Current Source  Initialize=on  Source_Type=AC  Amplitude=0  Phase=0  Frequency=0  Measurements=None
  Controlled Voltage Source : spsControlledVoltageSourceLib/Controlled Voltage Source  Initialize=on  Source_Type=AC  Amplitude=0  Phase=0  Frequency=0  Measurements=None
  Controlled Voltage Source1 : spsControlledVoltageSourceLib/Controlled Voltage Source  Initialize=on  Source_Type=AC  Amplitude=0  Phase=0  Frequency=0  Measurements=None
  Current Measurement : spsCurrentMeasurementLib/Current Measurement  PhasorSimulation=off  OutputType=Complex  PSBequivalent=0
  Current Measurement1 : spsCurrentMeasurementLib/Current Measurement  PhasorSimulation=off  OutputType=Complex  PSBequivalent=0
  Current Measurement2 : spsCurrentMeasurementLib/Current Measurement  PhasorSimulation=off  OutputType=Complex  PSBequivalent=0
  Demux1 : Demux  Outputs=3
      settings: DisplayOption=none
  Demux2 : Demux  Outputs=2
      settings: DisplayOption=none
  Gain : Gain
  Id computation : Subsystem
  Limit detection : Subsystem
  Mux : Mux  Inputs=2
  Mux2 : Mux  Inputs=3
  Mux4 : Mux  Inputs=2
  Output Resistance : spsThreePhaseSeriesRLCBranchLib/Three-Phase Series RLC Branch  LConnTagsString=A|B|C  RConnTagsString=A|B|C  BranchType=R  Resistance=100*Resistance  Inductance=1e-3  Capacitance=1e-6  Measurements=Branch voltages and currents
  Output Resistance correction : Subsystem
  Product1 : Product  RndMeth=Zero
  Sum : Sum  Inputs=|++
  Terminator : Terminator
  Unit Delay3 : UnitDelay  SampleTime=Ts  HasFrameUpgradeWarning=on
  Voltage Measurement : spsVoltageMeasurementLib/Voltage Measurement  PhasorSimulation=off  OutputType=Complex  PSBequivalent=0
  Voltage Measurement1 : spsVoltageMeasurementLib/Voltage Measurement  PhasorSimulation=off  OutputType=Complex  PSBequivalent=0
  Voltage Measurement3 : spsVoltageMeasurementLib/Voltage Measurement  PhasorSimulation=off  OutputType=Complex  PSBequivalent=0
  + : PMIOPort  Side=Right
  A : PMIOPort  Port=2  Side=Left
  B : PMIOPort  Port=3  Side=Left
  - : PMIOPort  Port=4  Side=Right
  C : PMIOPort  Port=5  Side=Left
  wires:
  Current Measurement/1 -> Mux2/1
  Current Measurement1/1 -> Mux2/2
  Voltage Measurement/1 -> Mux/1  "Vac"
  Voltage Measurement1/1 -> Mux/2  "Vbc"
  Mux/1 -> Mux4/2
  Current Measurement2/1 -> Mux2/3
  Mux4/1 -> Id computation/1(m)
  Mux2/1 -> Mux4/1  "Iabc"
  Id computation/1(Id) -> Controlled Current Source2/1
  Voltage Measurement3/1 -> Unit Delay3/1, Id computation/2(Vdc)
  Bus Selector1/1 -> Product1/2  "<Pulses*>"
  Demux1/1 -> Controlled Current Source/1
  Demux1/2 -> Controlled Current Source1/1
  Demux1/3 -> Terminator/1
  Demux2/2 -> Controlled Voltage Source1/1
  Demux2/1 -> Controlled Voltage Source/1
  Bus Selector2/1 -> Sum/1  "<iabc*>"
  Limit detection/1(Limit) -> Gain/1
  Sum/1 -> Demux1/1
  Unit Delay3/1 -> Product1/1, Limit detection/1(Vcc)
  ctrl/1 -> Bus Selector1/1, Limit detection/2(ctrl), Bus Selector2/1, Output Resistance correction/1(ctrl)
  Product1/1 -> Demux2/1  "Voltage*"
  Output Resistance correction/1("Iabc_r ") -> Sum/2
  Gain/1 -> Activation Switches/1(gate)
  connections:
  Voltage Measurement3/LConn1 -- Controlled Current Source2/LConn1 -- +/RConn1
  Voltage Measurement3/LConn2 -- Controlled Current Source2/RConn1 -- -/RConn1
  Activation Switches/LConn6 -- Controlled Current Source/LConn1 -- Controlled Current Source1/LConn1 -- Output Resistance/LConn3
  Output Resistance/RConn3 -- Output Resistance/RConn2 -- Output Resistance/RConn1
  Voltage Measurement/LConn1 -- Activation Switches/RConn1 -- Current Measurement/LConn1
  Output Resistance/LConn1 -- Activation Switches/LConn4 -- Controlled Current Source/RConn1
  Output Resistance/LConn2 -- Activation Switches/LConn5 -- Controlled Current Source1/RConn1
  Voltage Measurement/LConn2 -- Activation Switches/RConn3 -- Voltage Measurement1/LConn2 -- Current Measurement2/LConn1
  Controlled Voltage Source/LConn1 -- Activation Switches/LConn2 -- Controlled Voltage Source1/RConn1
  Voltage Measurement1/LConn1 -- Activation Switches/RConn2 -- Current Measurement1/LConn1
  Current Measurement/RConn1 -- A/RConn1
  Current Measurement1/RConn1 -- B/RConn1
  C/RConn1 -- Current Measurement2/RConn1
  Controlled Voltage Source/RConn1 -- Activation Switches/LConn1
  Activation Switches/LConn3 -- Controlled Voltage Source1/LConn1

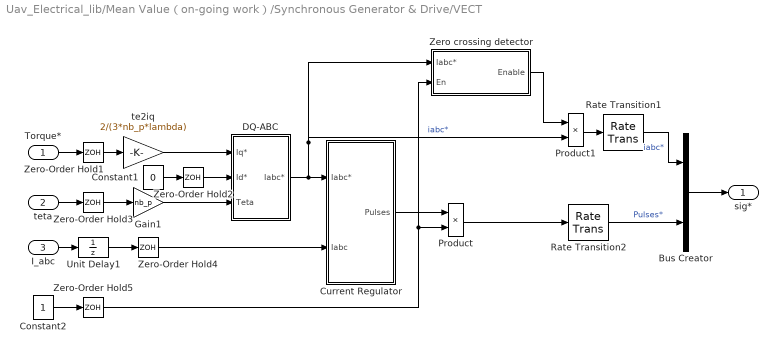
== system Uav_Electrical_lib/Mean Value（on-going work）/Synchronous Generator & Drive/VECT ==
  Torque* : Inport
  teta : Inport  Port=2
  I_abc : Inport  Port=3
  Bus Creator : BusCreator  Inputs=2
  Constant1 : Constant  Value=0
  Constant2 : Constant
  Current Regulator : Subsystem
  DQ-ABC : Subsystem
  Gain1 : Gain  Gain=nb_p  SaturateOnIntegerOverflow=on  OutDataTypeStr=Inherit: Same as input  ParamDataTypeStr=Inherit: Same as input
  Product : Product  RndMeth=Zero
  Product1 : Product  RndMeth=Zero
  Rate Transition1 : RateTransition
  Rate Transition2 : RateTransition
  Unit Delay1 : UnitDelay  SampleTime=Ts  HasFrameUpgradeWarning=on
  Zero crossing detector : Subsystem
  Zero-Order Hold{1..5} (5 alike) : ZeroOrderHold  SampleTime=Ts_vect
  te2iq : Gain  Gain=2/(3*nb_p*lambda)  SaturateOnIntegerOverflow=on  OutDataTypeStr=Inherit: Same as input  ParamDataTypeStr=Inherit: Same as input
  sig* : Outport  VectorParamsAs1DForOutWhenUnconnected=off
  wires:
  I_abc/1 -> Unit Delay1/1
  DQ-ABC/1(Iabc*) -> Current Regulator/1(Iabc*), Product1/2, Zero crossing detector/1(Iabc*)  "iabc*"
  Unit Delay1/1 -> Zero-Order Hold4/1
  Gain1/1 -> DQ-ABC/3(Teta)
  Constant1/1 -> Zero-Order Hold2/1
  Torque*/1 -> Zero-Order Hold1/1
  Zero-Order Hold3/1 -> Gain1/1
  teta/1 -> Zero-Order Hold3/1
  Zero-Order Hold1/1 -> te2iq/1
  Zero-Order Hold2/1 -> DQ-ABC/2("Id* ")
  te2iq/1 -> DQ-ABC/1("Iq* ")
  Bus Creator/1 -> sig*/1
  Rate Transition2/1 -> Bus Creator/2  "Pulses*"
  Rate Transition1/1 -> Bus Creator/1  "iabc*"
  Zero-Order Hold4/1 -> Current Regulator/2(Iabc)
  Current Regulator/1(Pulses) -> Product/1
  Product/1 -> Rate Transition2/1
  Product1/1 -> Rate Transition1/1
  Constant2/1 -> Zero-Order Hold5/1
  Zero crossing detector/1(Enable) -> Product1/1
  Zero-Order Hold5/1 -> Product/2, Zero crossing detector/2(En)

== system Uav_Electrical_lib/Mean Value（on-going work）/Synchronous Motor & Drive/GF ==
  In1 : Inport
  Out1 : Outport  VectorParamsAs1DForOutWhenUnconnected=off
  tag scope: Mot_TReq_SYS=global
  wires:
  In1/1 -> [Mot_TReq_SYS], Out1/1

== system Uav_Electrical_lib/Mean Value（on-going work）/Synchronous Motor & Drive/Measures ==
  Current Measurement : spsCurrentMeasurementLib/Current Measurement  Tag=PoWeRsYsTeMmEaSuReMeNt  PhasorSimulation=off  OutputType=Magnitude  PSBequivalent=0
      settings: AttributesFormatString=\n
  Current Measurement1 : spsCurrentMeasurementLib/Current Measurement  Tag=PoWeRsYsTeMmEaSuReMeNt  PhasorSimulation=off  OutputType=Magnitude  PSBequivalent=0
      settings: AttributesFormatString=\n
  Current Measurement2 : spsCurrentMeasurementLib/Current Measurement  Tag=PoWeRsYsTeMmEaSuReMeNt  PhasorSimulation=off  OutputType=Magnitude  PSBequivalent=0
      settings: AttributesFormatString=\n
  Mux1 : Mux  Inputs=3
  Ta : PMIOPort  Side=Left
  Tb : PMIOPort  Port=2  Side=Left
  Tc : PMIOPort  Port=3  Side=Left
  Mta : PMIOPort  Port=4  Side=Right
  Mtb : PMIOPort  Port=5  Side=Right
  Mtc : PMIOPort  Port=6  Side=Right
  I_abc : Outport  VectorParamsAs1DForOutWhenUnconnected=off
  wires:
  Current Measurement1/1 -> Mux1/2
  Current Measurement/1 -> Mux1/1
  Current Measurement2/1 -> Mux1/3
  Mux1/1 -> I_abc/1
  connections:
  Current Measurement1/RConn1 -- Mtb/RConn1
  Tb/RConn1 -- Current Measurement1/LConn1
  Current Measurement/RConn1 -- Mta/RConn1
  Ta/RConn1 -- Current Measurement/LConn1
  Tc/RConn1 -- Current Measurement2/LConn1
  Current Measurement2/RConn1 -- Mtc/RConn1

== system Uav_Electrical_lib/Mean Value（on-going work）/Synchronous Motor & Drive/Mux ==
  sig* : Inport
  m : Inport  Port=2
  Bus Creator : BusCreator  Inputs=2
  Ctrl : Outport  VectorParamsAs1DForOutWhenUnconnected=off
  wires:
  m/1 -> Bus Creator/2  "m"
  sig*/1 -> Bus Creator/1  "Signals*"
  Bus Creator/1 -> Ctrl/1

== system Uav_Electrical_lib/Mean Value（on-going work）/Synchronous Motor & Drive/Subsystem ==
  In1 : Inport
  "+ -> -1" : Gain  Gain=30/pi
  Bus Selector : BusSelector  OutputSignals=Stator current is_a (A),Rotor speed wm (rad/s),Electromagnetic torque Te (N*m)
  Mux1 : Mux  Inputs=2
  Mux2 : Mux  Inputs=3
  Motor : Outport  VectorParamsAs1DForOutWhenUnconnected=off
  tag scope: MotorDrive=global
  wires:
  Mux2/1 -> [MotorDrive]
  Bus Selector/1 -> Mux2/1  "<Stator current is_a (A)>"
  Mux1/1 -> Mux2/3
  Bus Selector/3 -> Mux1/1  "<Electromagnetic torque Te (N*m)>"
  Bus Selector/2 -> "+ -> -1"/1  "<Rotor speed wm (rad/s)>"
  [Mot_TReq_SYS] -> Mux1/2
  "+ -> -1"/1 -> Mux2/2
  In1/1 -> Motor/1, Bus Selector/1

== system Uav_Electrical_lib/Mean Value（on-going work）/Synchronous Motor & Drive/Subsystem1 ==
  Sig : Inport
  Bus Selector : BusSelector  OutputSignals=Electromagnetic torque Te (N*m)
  Ideal Rotational Motion Sensor : fl_lib/Mechanical/Mechanical Sensors/Ideal Rotational Motion Sensor  reference=foundation.enum.MeasurementReference.difference  acceleration_port=false  velocity_port=true  position_port=true  wrap_angle=simscape.enum.onoff.off  offset=0 rad
  Ideal Torque Source : fl_lib/Mechanical/Mechanical Sources/Ideal Torque Source
  Mechanical Rotational Reference : fl_lib/Mechanical/Rotational Elements/Mechanical Rotational Reference
  Mechanical Rotational Reference1 : fl_lib/Mechanical/Rotational Elements/Mechanical Rotational Reference
  PS-Simulink Converter : nesl_utility/PS-Simulink Converter  PhysicalDomain=network_engine_domain  SubClassName=ps_output  LeftPortType=input  RightPortType=output  PseudoPeriodic=off  Frequencies=[]  VectorFormat=1-D array  Unit=rad/s  AffineConversion=off
  Simulink-PS Converter : nesl_utility/Simulink-PS Converter  PhysicalDomain=network_engine_domain  SubClassName=ps_input  LeftPortType=input  RightPortType=output  PseudoPeriodic=off  Frequencies=[]  NoiseDistribution=none  NoiseParameters=[]  Unit=1  AffineConversion=off  FilteringAndDerivatives=zero  SimscapeFilterOrder=1  InputFilterTimeConstant=0.005  UdotUserProvided=0
  Sh : PMIOPort  Side=Right
  Spd : Outport  VectorParamsAs1DForOutWhenUnconnected=off
  wires:
  Bus Selector/1 -> Simulink-PS Converter/1  "<Electromagnetic torque Te (N*m)>"
  Sig/1 -> Bus Selector/1
  PS-Simulink Converter/1 -> Spd/1
  connections:
  Mechanical Rotational Reference/LConn1 -- Ideal Rotational Motion Sensor/RConn1
  Mechanical Rotational Reference1/LConn1 -- Ideal Torque Source/RConn2
  Ideal Torque Source/LConn1 -- Sh/RConn1 -- Ideal Rotational Motion Sensor/LConn1
  PS-Simulink Converter/LConn1 -- Ideal Rotational Motion Sensor/RConn2
  Simulink-PS Converter/RConn1 -- Ideal Torque Source/RConn1

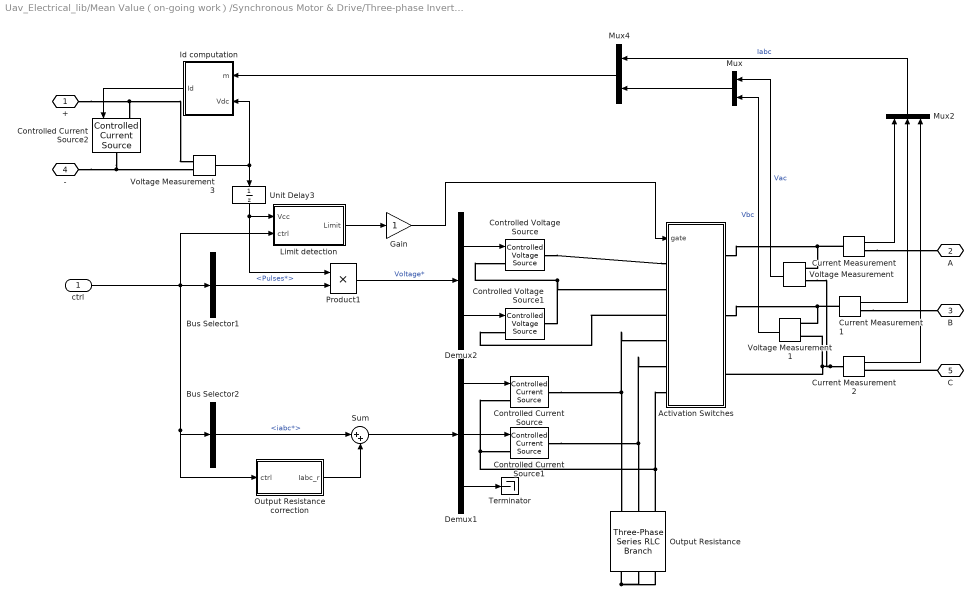
== system Uav_Electrical_lib/Mean Value（on-going work）/Synchronous Motor & Drive/Three-phase Inverter ==
  ctrl : Inport
  Activation Switches : Subsystem
  Bus Selector1 : BusSelector  OutputSignals=Signals*.Pulses*
  Bus Selector2 : BusSelector  OutputSignals=Signals*.iabc*
  Controlled Current Source : spsControlledCurrentSourceLib/Controlled Current Source  Initialize=on  Source_Type=AC  Amplitude=0  Phase=0  Frequency=0  Measurements=None
  Controlled Current Source1 : spsControlledCurrentSourceLib/Controlled Current Source  Initialize=on  Source_Type=AC  Amplitude=0  Phase=0  Frequency=0  Measurements=None
  Controlled Current Source2 : spsControlledCurrentSourceLib/Controlled Current Source  Initialize=on  Source_Type=AC  Amplitude=0  Phase=0  Frequency=0  Measurements=None
  Controlled Voltage Source : spsControlledVoltageSourceLib/Controlled Voltage Source  Initialize=on  Source_Type=AC  Amplitude=0  Phase=0  Frequency=0  Measurements=None
  Controlled Voltage Source1 : spsControlledVoltageSourceLib/Controlled Voltage Source  Initialize=on  Source_Type=AC  Amplitude=0  Phase=0  Frequency=0  Measurements=None
  Current Measurement : spsCurrentMeasurementLib/Current Measurement  PhasorSimulation=off  OutputType=Complex  PSBequivalent=0
  Current Measurement1 : spsCurrentMeasurementLib/Current Measurement  PhasorSimulation=off  OutputType=Complex  PSBequivalent=0
  Current Measurement2 : spsCurrentMeasurementLib/Current Measurement  PhasorSimulation=off  OutputType=Complex  PSBequivalent=0
  Demux1 : Demux  Outputs=3
      settings: DisplayOption=none
  Demux2 : Demux  Outputs=2
      settings: DisplayOption=none
  Gain : Gain
  Id computation : Subsystem
  Limit detection : Subsystem
  Mux : Mux  Inputs=2
  Mux2 : Mux  Inputs=3
  Mux4 : Mux  Inputs=2
  Output Resistance : spsThreePhaseSeriesRLCBranchLib/Three-Phase Series RLC Branch  LConnTagsString=A|B|C  RConnTagsString=A|B|C  BranchType=R  Resistance=100*Resistance  Inductance=1e-3  Capacitance=1e-6  Measurements=Branch voltages and currents
  Output Resistance correction : Subsystem
  Product1 : Product  RndMeth=Zero
  Sum : Sum  Inputs=|++
  Terminator : Terminator
  Unit Delay3 : UnitDelay  SampleTime=Ts  HasFrameUpgradeWarning=on
  Voltage Measurement : spsVoltageMeasurementLib/Voltage Measurement  PhasorSimulation=off  OutputType=Complex  PSBequivalent=0
  Voltage Measurement1 : spsVoltageMeasurementLib/Voltage Measurement  PhasorSimulation=off  OutputType=Complex  PSBequivalent=0
  Voltage Measurement3 : spsVoltageMeasurementLib/Voltage Measurement  PhasorSimulation=off  OutputType=Complex  PSBequivalent=0
  + : PMIOPort  Side=Right
  A : PMIOPort  Port=2  Side=Left
  B : PMIOPort  Port=3  Side=Left
  - : PMIOPort  Port=4  Side=Right
  C : PMIOPort  Port=5  Side=Left
  wires:
  Output Resistance correction/1("Iabc_r ") -> Sum/2
  Id computation/1(Id) -> Controlled Current Source2/1
  Gain/1 -> Activation Switches/1(gate)
  Product1/1 -> Demux2/1  "Voltage*"
  ctrl/1 -> Output Resistance correction/1(ctrl), Bus Selector2/1, Limit detection/2(ctrl), Bus Selector1/1
  Unit Delay3/1 -> Limit detection/1(Vcc), Product1/1
  Sum/1 -> Demux1/1
  Limit detection/1(Limit) -> Gain/1
  Bus Selector2/1 -> Sum/1  "<iabc*>"
  Demux2/1 -> Controlled Voltage Source/1
  Demux2/2 -> Controlled Voltage Source1/1
  Demux1/3 -> Terminator/1
  Demux1/2 -> Controlled Current Source1/1
  Demux1/1 -> Controlled Current Source/1
  Bus Selector1/1 -> Product1/2  "<Pulses*>"
  Voltage Measurement3/1 -> Id computation/2(Vdc), Unit Delay3/1
  Mux2/1 -> Mux4/1  "Iabc"
  Mux4/1 -> Id computation/1(m)
  Current Measurement2/1 -> Mux2/3
  Mux/1 -> Mux4/2
  Voltage Measurement1/1 -> Mux/2  "Vbc"
  Voltage Measurement/1 -> Mux/1  "Vac"
  Current Measurement1/1 -> Mux2/2
  Current Measurement/1 -> Mux2/1
  connections:
  Activation Switches/LConn3 -- Controlled Voltage Source1/LConn1
  Controlled Voltage Source/RConn1 -- Activation Switches/LConn1
  C/RConn1 -- Current Measurement2/RConn1
  Current Measurement1/RConn1 -- B/RConn1
  Current Measurement/RConn1 -- A/RConn1
  Current Measurement1/LConn1 -- Activation Switches/RConn2 -- Voltage Measurement1/LConn1
  Controlled Voltage Source1/RConn1 -- Activation Switches/LConn2 -- Controlled Voltage Source/LConn1
  Current Measurement2/LConn1 -- Voltage Measurement1/LConn2 -- Activation Switches/RConn3 -- Voltage Measurement/LConn2
  Controlled Current Source1/RConn1 -- Activation Switches/LConn5 -- Output Resistance/LConn2
  Controlled Current Source/RConn1 -- Activation Switches/LConn4 -- Output Resistance/LConn1
  Current Measurement/LConn1 -- Activation Switches/RConn1 -- Voltage Measurement/LConn1
  Output Resistance/RConn1 -- Output Resistance/RConn2 -- Output Resistance/RConn3
  Output Resistance/LConn3 -- Controlled Current Source1/LConn1 -- Controlled Current Source/LConn1 -- Activation Switches/LConn6
  -/RConn1 -- Controlled Current Source2/RConn1 -- Voltage Measurement3/LConn2
  +/RConn1 -- Controlled Current Source2/LConn1 -- Voltage Measurement3/LConn1

== system Uav_Electrical_lib/Mean Value（on-going work）/Synchronous Motor & Drive/Torque limitation ==
  N rad/s : Inport
  Torque : Inport  Port=2
  Abs1 : Abs
  Gain : Gain  Gain=-1
  Saturation Dynamic : simulink/Discontinuities/Saturation Dynamic  OutMin=[]  OutMax=[]  OutDataTypeStr=Inherit: Same as second input  OutDataType=sfix(16)  OutScaling=2^-10  DoSatur=off
  Torque vs speed profile : Lookup  InputValues=uavParams.MotorElec.TorqSpdLUT.SpeedRPM*pi/30  Table=uavParams.MotorElec.TorqSpdLUT.TorqueNm  SaturateOnIntegerOverflow=off
  torque : Outport  VectorParamsAs1DForOutWhenUnconnected=off
  wires:
  Gain/1 -> Saturation Dynamic/3
  Torque/1 -> Saturation Dynamic/2
  Saturation Dynamic/1 -> torque/1
  Torque vs speed profile/1 -> Gain/1, Saturation Dynamic/1
  Abs1/1 -> Torque vs speed profile/1
  N rad/s/1 -> Abs1/1
